simulink model "modeChanger"  (R2020a)
settings: Solver=FixedStepAuto  StartTime=0.0  StopTime=inf  FixedStep=0.02  RelTol=1e-3
libraries: robotlib x7
settings Model: Creator=sprinkle  LastModifiedBy=ivory
settings OptimizationCC: UseFloatMulNetSlope=on  EnhancedBackFolding=on  EfficientFloat2IntCast=on  MaxStackSize=64  OptimizeBlockOrder=speed  DifferentSizesBufferReuse=on  OptimizationCustomize=off  EfficientTunableParamExpr=on
settings DebuggingCC: ParameterTunabilityLossMsg=error
settings HardwareCC: ProdBitPerPointer=32  ProdBitPerSizeT=32  ProdBitPerPtrDiffT=32  ProdLargestAtomicFloat=None  ProdIntDivRoundTo=Undefined  ProdEndianess=Unspecified  ProdWordSize=32  ProdHWDeviceType=Generic->Unspecified (assume 32-bit Generic)  UseEmbeddedCoderFeatures=off
settings SFSimCC: MATLABDynamicMemAlloc=off
settings RTWCC: SystemTargetFile=ert.tlc  HardwareBoard=Robot Operating System (ROS)  TemplateMakefile=ert_default_tmf  GenerateReport=on  Toolchain=Catkin  BuildConfiguration=Faster Runs  LaunchReport=on  TargetLang=C++
settings CodeAppCC: ForceParamTrailComments=on  OperatorAnnotations=on
settings ERTTargetCC: ERTCustomFileBanners=off  SupportNonFinite=off  SupportContinuousTime=on  SupportNonInlinedSFcns=on  ModelStepFunctionPrototypeControlCompliant=off  RootIOFormat=Structure reference

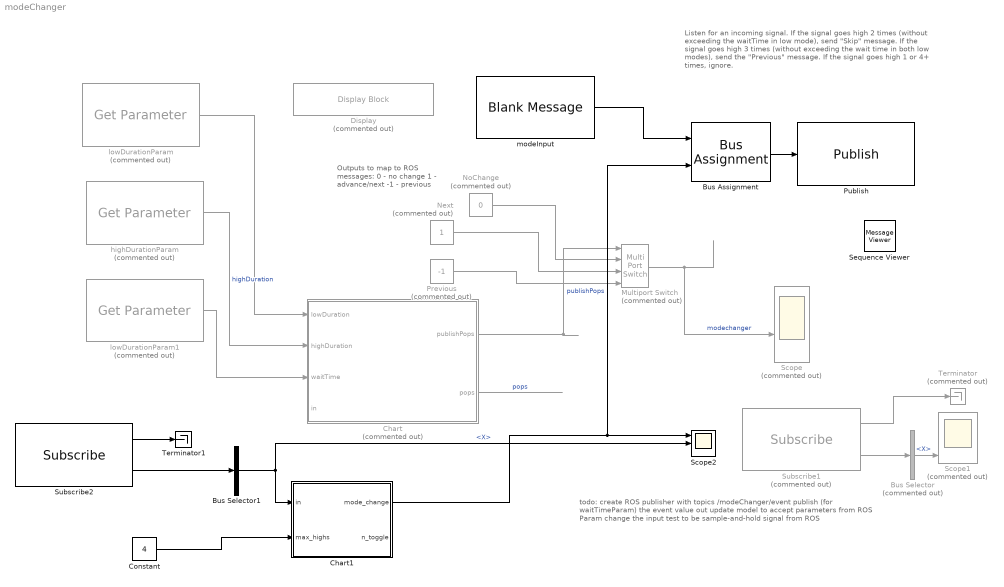
== system modeChanger ==
  note: todo:
      | create ROS publisher with topics /modeChanger/event
      | publish (for waitTimeParam) the event value out
      | update model to accept parameters from ROS Param
      | change the input test to be sample-and-hold signal from ROS
  note: Listen for an incoming signal. If the signal goes high 2 times (without exceeding the waitTime in low mode), send "Skip" message. If the signal goes high 3 times (without exceeding the wait time in both low modes), send the "Previous" message. If the signal goes high 1 or 4+ times, ignore.
  note: Outputs to map to ROS messages:
      | 0 - no change
      | 1 - advance/next
      | -1 - previous
  Bus Assignment : BusAssignment  AssignedSignals=Data
  Bus Selector : BusSelector  Commented=on  DialogController=Simulink.DDGSource_BusSelector  OutputSignals=Linear.X
  Bus Selector1 : BusSelector  DialogController=Simulink.DDGSource_BusSelector  OutputSignals=Linear.X
  Chart : Stateflow chart  Commented=on  TreatAsAtomicUnit=on
  Chart1 : Stateflow chart  TreatAsAtomicUnit=on
  Constant : Constant  Value=4
  Display : DisplayBlock  Commented=on  LabelPosition=Hide  Format=short  Transparency=1
  Multiport Switch : MultiPortSwitch  Commented=on  DataPortOrder=Specify indices  DataPortIndices={0,2,3}
  Next : Constant  Commented=on  OutDataTypeStr=int8
  NoChange : Constant  Commented=on  Value=0  OutDataTypeStr=int8
  Previous : Constant  Commented=on  Value=-1  OutDataTypeStr=int8
  Publish : robotlib/Publish  topicSource=Specify your own  topic=/modeChanger  messageType=std_msgs/Int8  messageQueueLength=1
  Scope : Scope  Commented=on  NumInputPorts=4
  Scope1 : Scope  Commented=on  NumInputPorts=4
  Scope2 : Scope  NumInputPorts=3
  Sequence Viewer : MessageViewer  History=1000  SavedRootId=#
  Subscribe1 : robotlib/Subscribe  Commented=on  topicSource=Specify your own  topic=modeChanger  messageType=geometry_msgs/Twist  sampleTime=0.05  messageQueueLength=1
  Subscribe2 : robotlib/Subscribe  topicSource=Specify your own  topic=/highbeams  messageType=geometry_msgs/Twist  sampleTime=-1  messageQueueLength=1
  Terminator : Terminator  Commented=on
  Terminator1 : Terminator
  highDurationParam : robotlib/Get Parameter  Commented=on  ParameterSource=Specify your own  ParameterName=/highDuration  ParameterType=double  ParameterMaxArrayLength=16  ParameterInitialValue=0.05  SampleTime=-1  ShowErrorCodeOutput=off  ModelName=modeChanger  BlockId=ParamGet_modeChanger_59
      settings: SourceProductBaseCode=RR
  lowDurationParam : robotlib/Get Parameter  Commented=on  ParameterSource=Specify your own  ParameterName=/lowDuration  ParameterType=double  ParameterMaxArrayLength=16  ParameterInitialValue=0.05  SampleTime=-1  ShowErrorCodeOutput=off  ModelName=modeChanger  BlockId=ParamGet_modeChanger_56
      settings: SourceProductBaseCode=RR
  lowDurationParam1 : robotlib/Get Parameter  Commented=on  ParameterSource=Specify your own  ParameterName=/waitTime  ParameterType=double  ParameterMaxArrayLength=16  ParameterInitialValue=0.35  SampleTime=-1  ShowErrorCodeOutput=off  ModelName=modeChanger  BlockId=ParamGet_modeChanger_60
      settings: SourceProductBaseCode=RR
  modeInput : robotlib/Blank Message  messageClass=Message  entityType=std_msgs/Int8  messageType=std_msgs/Int8  SampleTime=-1
  wires:
  highDurationParam/1 -> Chart/2(highDuration)  "highDuration"
  Subscribe2/2 -> Bus Selector1/1
  Previous/1 -> Multiport Switch/4
  Next/1 -> Multiport Switch/3
  Multiport Switch/1 -> Scope/3  "modechanger"
  NoChange/1 -> Multiport Switch/2
  Bus Assignment/1 -> Publish/1
  modeInput/1 -> Bus Assignment/1
  Subscribe1/1 -> Terminator/1
  Subscribe1/2 -> Bus Selector/1
  Bus Selector/1 -> Scope1/4  "<X>"
  Subscribe2/1 -> Terminator1/1
  Bus Selector1/1 -> Scope2/2, Chart1/1(in)  "<X>"
  lowDurationParam/1 -> Chart/1(lowDuration)
  lowDurationParam1/1 -> Chart/3(waitTime)
  Chart/2(pops) -> ?  "pops"
  Chart/1(publishPops) -> Multiport Switch/1  "publishPops"
  Chart1/1(mode_change) -> Scope2/1, Bus Assignment/2
  Constant/1 -> Chart1/2(max_highs)
  ? -> Scope2/3

== stateflow chart modeChanger/Chart ==
  state ResetPops
    entry: pops=0;
  state Reset
  state idle
  state HeldIn
  state initialize
    entry: pops=0
  state High
  state Pop
    entry: pops=pops+1;
  state Debounce
  Reset -> ResetPops [order 2] : [pops<=1]
  ResetPops -> idle : after(waitTime,sec){publishPops=0;}
  Reset -> ResetPops [order 1] : [pops>1]{publishPops=pops;}
  idle -> Reset [order 2] : after(waitTime,sec)
  Pop -> idle [order 1] : [pops<=3]
  initialize -> idle
  (default) -> initialize
  HeldIn -> idle : [in==0]{pops=0;}
  High -> idle [order 1] : [in==0]
  idle -> High [order 1] : [in>0]{publishPops=0;}
  Pop -> HeldIn [order 2] : [pops>3]
  Debounce -> HeldIn [order 1] : after(waitTime,sec)
  High -> Debounce [order 2] : after(highDuration,sec)
  Debounce -> Pop [order 2] : [in==0]
  data: lowDuration input; highDuration input; waitTime input; in input; publishPops output int8; pops output int8

== stateflow chart modeChanger/Chart1 ==
  note: Treat low (high)^n low as low high low for some n less than a certain value max_highs
  state high_after_high
    entry:
    n_high = n_high + 1;
  state mode_change_1
    entry: mode_change = 1;
  state high
    entry: n_high = 1;
  state Initialize
    entry: n_toggle = 0;
  state Idle
    entry: n_high = 0;
  state mode_change_minus1
    entry: mode_change  = -1;
  state low
    entry: n_low = 0;
    n_toggle = 0;
  state low_after_high
    entry: n_toggle = n_toggle + 1;
    n_high = 0;
  state high_after_low
    entry: n_low = 0;
  state low_after_low
    entry: n_low = n_low + 1;
    mode_change = 0;
  state mode_change_0
    entry: mode_change = 0;
  high_after_low -> high_after_high [order 2] : [in == 1]
  mode_change_1 -> low_after_low [order 1] : [in == 0]
  high_after_high -> high_after_high [order 2] : [in == 1]
  high -> high_after_high [order 1] : [in == 1]
  high_after_high -> low [order 1] : [in == 0]
  Idle -> high [order 2] : [in == 1]
  (default) -> Initialize
  high -> low [order 2] : [in == 0]
  mode_change_1 -> high_after_low [order 2] : [in ==1]
  low_after_high -> mode_change_1 [order 1] : [n_toggle == 2]
  mode_change_minus1 -> low_after_low [order 1] : [in == 0]
  Initialize -> Idle
  Idle -> low [order 1] : [in == 0]
  mode_change_minus1 -> high_after_low [order 2] : [in == 1]
  low_after_high -> mode_change_minus1 [order 2] : [n_toggle == 3]
  low -> high_after_low [order 1] : [in == 1]
  low -> low_after_high [order 3] : [n_high < max_highs]
  low -> low_after_low [order 2] : [in == 0]
  low_after_high -> mode_change_0 [order 3] : [n_toggle > 3 || n_toggle < 2]
  low_after_low -> low_after_low [order 2] : [in == 0]
  high_after_low -> low_after_high [order 1] : [in == 0]
  low_after_low -> high_after_low [order 1] : [in == 1]
  mode_change_0 -> high_after_low [order 2] : [in == 1]
  mode_change_0 -> low_after_low [order 1] : [in == 0]
  data: mode_change output int8; in input; max_highs input; n_high local; n_toggle output
